simulink model "sample_overview"  (R2022a)
settings: configuration reference "MainConfig" (kept outside this file)
PostLoadFcn:
  | load('input_modelo_bateria.mat')
undefined symbols (not defined in the file or in its folder): rest_time, SOC_MAX, SOC_MIN, Temperature
libraries: fl_lib x1, nesl_utility x1
settings Model: PacingRate=1000  Creator=eduardo.guimaraes  LastModifiedBy=mateu
settings ConfigSetRef: SourceName=MainConfig  SourceLocation=Base Workspace

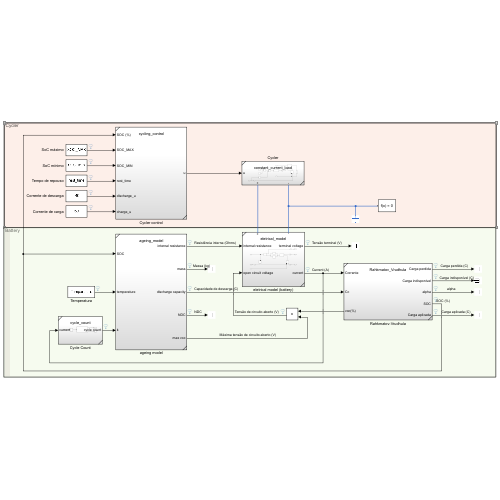
[thumbnail: Simulink's stored preview of the top-level diagram]
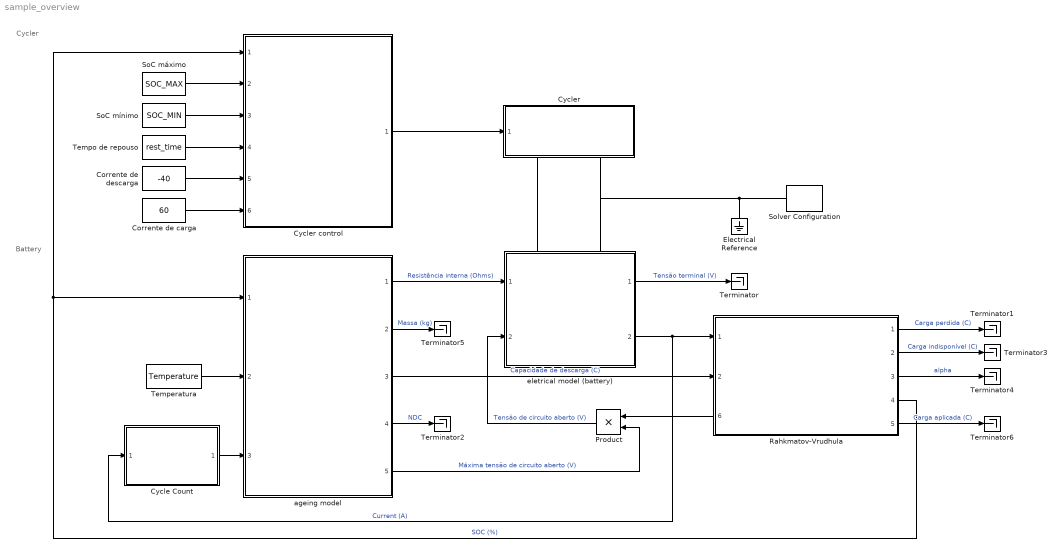
== system sample_overview ==
  note: Cycler
  note: Battery
  Corrente de carga : Constant  Value=60
  Corrente de descarga : Constant  Value=-40
  Cycle Count : Subsystem  ReferencedSubsystem=cycle_count
  Cycler : Subsystem  ReferencedSubsystem=constant_current_load
      settings: PortSchema="{\"entries\":[{\"content\":{\"sides\":[{\"content\":{\"connectorIds\":[\"In1\"]},\"type\":\"ConnectorPlacement.EquallySpacedRectSide\",\"uuid\":\"1f5119c1-e4c4-4d36-9ce4-0a74503307ce\"},{\"content\":{\"connectorIds\":[],\"side\":\"RIGHT\"},\"type\":\"ConnectorPlacement.EquallySpacedRectSide\",\"uuid\":\"dcdfbcd6-0df9-4737-b1f4-f8955107c991\"},{\"content\":{\"connectorIds\":[],\"side\":\"TOP\"},\"type\":\"ConnectorPlacement.EquallySpacedRectSide\",\"uuid\":\"b6d21308-5cb8-408e-91b8-1a923178fca9\"},{\"content\":{\"connectorIds\":[\"RConn1\",\"RConn2\"],\"side\":\"BOTTOM\"},\"type\":\"ConnectorPlacement.EquallySpacedRectSide\",\"uuid\":\"e4f630e3-91bb-4100-954f-0aef13f842b9\"}]},\"type\":\"ConnectorPlacement.EquallySpacedConnector\",\"uuid\":\"c9fbcd82-4c46-4ddd-ab65-01b0bdfa28a4\"}],\"packageUris\":[\"http://schema.mathworks.com/mf0/Connector/R2020b\"],\"version\":\"1.0\"}"
  Cycler control : Subsystem  ReferencedSubsystem=cycling_control
  Electrical Reference : fl_lib/Electrical/Electrical Elements/Electrical Reference
      settings: SourceProductBaseCode=PW,SS,VE
  Product : Product
  Rahkmatov-Vrudhula : Subsystem  ReferencedSubsystem=Rahkmatov_Vrudhula
      settings: PortSchema="{\"entries\":[{\"content\":{\"sides\":[{\"content\":{\"connectorIds\":[\"In1\",\"In2\",\"Out6\"]},\"type\":\"ConnectorPlacement.EquallySpacedRectSide\",\"uuid\":\"83f3e873-db9f-47d1-b7c3-7eda48a10b32\"},{\"content\":{\"connectorIds\":[\"Out1\",\"Out2\",\"Out3\",\"Out4\",\"Out5\"],\"side\":\"RIGHT\"},\"type\":\"ConnectorPlacement.EquallySpacedRectSide\",\"uuid\":\"48ac6012-cdb4-4752-bc48-afa50bea9f0a\"},{\"content\":{\"connectorIds\":[],\"side\":\"TOP\"},\"type\":\"ConnectorPlacement.EquallySpacedRectSide\",\"uuid\":\"9cdc78bf-a718-48f1-92e6-e4070151caee\"}]},\"type\":\"ConnectorPlacement.EquallySpacedConnector\",\"uuid\":\"a231f58d-8e16-4cb4-bc80-61541bcf90eb\"}],\"packageUris\":[\"http://schema.mathworks.com/mf0/Connector/R2020b\"],\"version\":\"1.0\"}"
  SoC máximo : Constant  Value=SOC_MAX
  SoC mínimo : Constant  Value=SOC_MIN
  Solver Configuration : nesl_utility/Solver Configuration  PhysicalDomain=network_engine_domain  SubClassName=solver  LeftPortType=input  RightPortType=generic  Tones=[]  Harmonics=[]  SimulateNoise=off  Profile=off  UseLocalSampling=off  EnableSwitchedLinearOptims=on  FrequencyDomain=off  UseCCode=off  RelTol=0.001  AbsTol=0.001  MinStep=1e-09  ToWorkspace=off  RevertToSquareIcSolve=off  NumHomotopyIterations=100  PhasorMode=off  PhasorModeNumHarmonics=1  IndexReductionMethod=DerivativeReplacement  DoDC=off  ResidualTolerance=1e-09  UseLocalSolver=off  LocalSolverChoice=NE_BACKWARD_EULER_ADVANCER  LocalSolverSampleTime=0.001  DoFixedCost=off  MaxNonlinIter=3  MaxModeIter=2  ComputeImpulses=off  ImpulseIterations=2  LinearAlgebra=auto  LinearAlgebraNumThread=0  EquationFormulation=NE_TIME_EF  DelaysMemoryBudget=1024  AutomaticFiltering=on  FilteringTimeConstant=0.001  PartitionStorageMethod=AS_NEEDED  PartitionMemoryBudget=1024  PartitionMethod=ROBUST
      settings: SourceProductBaseCode=SS,PW,VE
  Temperatura : Constant  Value=Temperature
  Tempo de repouso : Constant  Value=rest_time
  Terminator{,1..6} (7 alike) : Terminator
  ageing model : Subsystem  ReferencedSubsystem=ageing_model
  eletrical model (battery) : Subsystem  ReferencedSubsystem=eletrical_model
      settings: PortSchema="{\"entries\":[{\"content\":{\"sides\":[{\"content\":{\"connectorIds\":[\"In1\",\"In2\"]},\"type\":\"ConnectorPlacement.EquallySpacedRectSide\",\"uuid\":\"e6309cc0-43d6-42db-b46d-fb5b38de698a\"},{\"content\":{\"connectorIds\":[\"Out1\",\"Out2\"],\"side\":\"RIGHT\"},\"type\":\"ConnectorPlacement.EquallySpacedRectSide\",\"uuid\":\"a3175445-87c0-47b1-a387-288225673634\"},{\"content\":{\"connectorIds\":[\"LConn1\",\"LConn2\"],\"side\":\"TOP\"},\"type\":\"ConnectorPlacement.EquallySpacedRectSide\",\"uuid\":\"f4aa44c9-f4dc-4aa8-a833-4f30710d8785\"},{\"content\":{\"connectorIds\":[],\"side\":\"BOTTOM\"},\"type\":\"ConnectorPlacement.EquallySpacedRectSide\",\"uuid\":\"f1117e0f-3189-4255-ad3f-4e2c31bb9482\"}]},\"type\":\"ConnectorPlacement.EquallySpacedConnector\",\"uuid\":\"e93a8d23-5e48-4dda-985c-f45f4ee27765\"}],\"packageUris\":[\"http://schema.mathworks.com/mf0/Connector/R2020b\"],\"version\":\"1.0\"}"
  wires:
  ageing model/3 -> Rahkmatov-Vrudhula/2  "Capacidade de descarga (C)"
  SoC máximo/1 -> Cycler control/2
  SoC mínimo/1 -> Cycler control/3
  eletrical model (battery)/2 -> Cycle Count/1, Rahkmatov-Vrudhula/1  "Current (A)"
  ageing model/1 -> eletrical model (battery)/1  "Resistência interna (Ohms)"
  Rahkmatov-Vrudhula/6 -> Product/1
  ageing model/5 -> Product/2  "Máxima tensão de circuito aberto (V)"
  Product/1 -> eletrical model (battery)/2  "Tensão de circuito aberto (V)"
  eletrical model (battery)/1 -> Terminator/1  "Tensão terminal (V)"
  Rahkmatov-Vrudhula/1 -> Terminator1/1  "Carga perdida (C)"
  Rahkmatov-Vrudhula/2 -> Terminator3/1  "Carga indisponível (C)"
  Rahkmatov-Vrudhula/3 -> Terminator4/1  "alpha"
  ageing model/4 -> Terminator2/1  "NDC"
  ageing model/2 -> Terminator5/1  "Massa (kg)"
  Rahkmatov-Vrudhula/5 -> Terminator6/1  "Carga aplicada (C)"
  Cycler control/1 -> Cycler/1
  Tempo de repouso/1 -> Cycler control/4
  Rahkmatov-Vrudhula/4 -> Cycler control/1, ageing model/1  "SOC (%)"
  Cycle Count/1 -> ageing model/3
  Temperatura/1 -> ageing model/2
  Corrente de carga/1 -> Cycler control/6
  Corrente de descarga/1 -> Cycler control/5
  connections:
  Electrical Reference/LConn1 -- eletrical model (battery)/LConn2 -- Cycler/RConn2 -- Solver Configuration/RConn1
  Cycler/RConn1 -- eletrical model (battery)/LConn1
